simulink model "testBeam"  (R2014a)
settings: Solver=ode23t  StartTime=0.0  StopTime=100  MaxStep=1  RelTol=1e-3  AbsTol=1e-3
PreLoadFcn:
  | K = 1e6;
  | C = 1e4;
  | L = 1;
  | w = 0.5;
  | d = 0.1;
undefined symbols (not defined in the file): X, Y, Z
libraries: beamLib x25, sm_lib x7, nesl_utility x3, simulink x1
settings Model: Creator=grouleau  LastModifiedBy=grouleau
settings SolverCC: MaxConsecutiveZCs=100  SolverJacobianMethodControl=SparsePerturbation  ZeroCrossAlgorithm=Adaptive
settings DebuggingCC: UnderspecifiedInitializationDetection=Classic  ParameterPrecisionLossMsg=none
settings SimscapeCC: SimscapeLogType=all  SimscapeLogSimulationStatistics=on  SimscapeLogLimitData=off
settings ExplorerConfigSet: InternalSimMechanicsExplorerSettings="<ExplorerConfiguration><canonicalview>default</canonicalview><AnimationSetting><BasePlaybackSpeed>1.0</BasePlaybackSpeed><PlaybackSpeedFactor>8.0</PlaybackSpeedFactor></AnimationSetting><TilePanel><TileInfo><Tiles Columns=\"1\" Count=\"1\" Rows=\"1\"><Column Left=\"2\" Weight=\"1\"/><Column Left=\"828\"/><Row Top=\"2\" Weight=\"1\"/><Row Top=\"712\"/><Tile Height=\"1\" Width=\"1\" X=\"0\" Y=\"0\"/></Tiles></TileInfo><SceneInfo><SceneViewer><BGColor><R>0.60000002384185791</R><G>0.60000002384185791</G><B>0.60000002384185791</B></BGColor><Camera><Position><X>12.490758895874023</X><Y>0.67244863510131836</Y><Z>26.566392370959054</Z></Position><Center><X>12.490758895874023</X><Y>0.67244863510131836</Y><Z>0</Z></Center><Up><X>0</X><Y>1</Y><Z>-0</Z></Up><Left>-13.115296840667725</Left><Right>13.115296840667725</Right><Bottom>-0.91037138700485232</Bottom><Top>0.91037138700485232</Top></Camera></SceneViewer></SceneInfo></TilePanel></ExplorerConfiguration>"

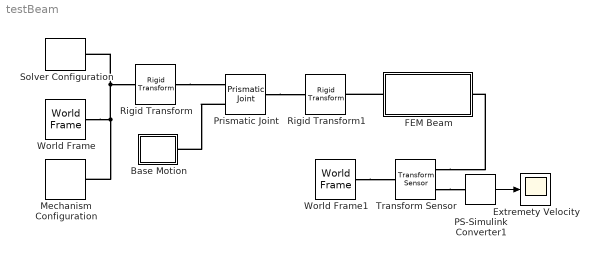
== system testBeam ==
  Base Motion : Subsystem
  Extremety Velocity : Scope
      settings: YMin=-50  YMax=50
  FEM Beam : Subsystem  mask{K=K, C=C, L=L, w=w, d=d, N=25}
      mask prompts: K "Stiffness"; C "Damping"; L "Length"; w "width"; d "Tickness"; N "Numbe rof elements"
      mask init:
      | blk = gcb;
      | 
      | blks = find_system(blk,'lookundermasks','all',...
      |     'followlinks','on',...
      |     'findall','on');
      | 
      | [hB, hF] = delete_beam_segments(blks);
      | add_beam_segments(blk,hB,hF,N)
  Mechanism Configuration : sm_lib/Utilities/Mechanism Configuration  UniformGravity=Constant  GravityVector=[0 0 -9.80665]*0  GravityUnits=m/s^2  LinearizationDelta=0.001  BlockFunction=simmechanics.library.utilities.mechanism_configuration
  PS-Simulink Converter1 : nesl_utility/PS-Simulink Converter  PhysicalDomain=network_engine_domain  SubClassName=ps_output  LeftPortType=input  RightPortType=output  PseudoPeriodic=off  Frequencies=[]  Unit=1  AffineConversion=off
  Prismatic Joint : sm_lib/Joints/Prismatic Joint  SenseConstraintForce=off  SenseConstraintForceX=off  SenseConstraintForceY=off  SenseConstraintForceZ=off  SenseConstraintTorque=off  SenseConstraintTorqueX=off  SenseConstraintTorqueY=off  SenseConstraintTorqueZ=off  SenseTotalForce=off  SenseTotalForceX=off  SenseTotalForceY=off  SenseTotalForceZ=off  SenseTotalTorque=off  SenseTotalTorqueX=off  SenseTotalTorqueY=off  SenseTotalTorqueZ=off  CompositeWrenchDir=FollowerOnBase  CompositeWrenchFrame=BaseFrame  EquilibriumPosition=0  EquilibriumPositionUnits=m  SpringStiffness=0  SpringStiffnessUnits=N/m  DampingCoefficient=0  DampingCoefficientUnits=N/(m/s)  TorqueActuationMode=ComputedTorque  MotionActuationMode=InputMotion  SensePosition=off  SenseVelocity=off  SenseAcceleration=off  SenseTorqueForce=off  PositionTargetValue=0  PositionTargetValueUnits=m  PositionTargetSpecify=off  PositionTargetPriority=High  VelocityTargetValue=0  VelocityTargetValueUnits=m/s  VelocityTargetSpecify=off  VelocityTargetPriority=High  BlockFunction=simmechanics.library.joints.prismatic_joint
  Rigid Transform : sm_lib/Frames and Transforms/Rigid Transform  TranslationMethod=None  TranslationLengthUnit=m  TranslationStandardAxis=+Z  TranslationStandardOffset=0  TranslationCartesianOffset=[0 0 0]  TranslationROffset=0  TranslationROffsetUnits=m  TranslationZOffset=0  TranslationZOffsetUnits=m  TranslationThetaOffset=0  TranslationThetaOffsetUnits=deg  RotationMethod=StandardAxis  RotationAngleUnits=deg  RotationStandardAxis=+X  RotationAngle=-90  RotationArbitraryAxis=[0 0 1]  FollAlignAxisA=+X  BaseAlignAxisA=+Y  FollAlignAxisB=+Y  BaseAlignAxisB=+Z  BlockFunction=simmechanics.library.frames_transforms.rigid_transform
  Rigid Transform1 : sm_lib/Frames and Transforms/Rigid Transform  TranslationMethod=None  TranslationLengthUnit=m  TranslationStandardAxis=+Z  TranslationStandardOffset=0  TranslationCartesianOffset=[0 0 0]  TranslationROffset=0  TranslationROffsetUnits=m  TranslationZOffset=0  TranslationZOffsetUnits=m  TranslationThetaOffset=0  TranslationThetaOffsetUnits=deg  RotationMethod=StandardAxis  RotationAngleUnits=deg  RotationStandardAxis=+X  RotationAngle=-90  RotationArbitraryAxis=[0 0 1]  FollAlignAxisA=+X  BaseAlignAxisA=+Y  FollAlignAxisB=+Y  BaseAlignAxisB=+Z  BlockFunction=simmechanics.library.frames_transforms.rigid_transform
  Solver Configuration : nesl_utility/Solver Configuration  PhysicalDomain=network_engine_domain  SubClassName=solver  LeftPortType=input  RightPortType=generic  Accelerate=off  Tones=[]  Harmonics=[]  SimulateNoise=off  Profile=off  UseLocalSampling=off  EnableSwitchedLinearOptims=on  FrequencyDomain=off  UseCCode=off  RelTol=0.001  AbsTol=1e-06  MinStep=1e-09  ToWorkspace=off  DoDC=off  ResidualTolerance=1e-09  UseLocalSolver=off  LocalSolverChoice=NE_BACKWARD_EULER_ADVANCER  LocalSolverSampleTime=0.001  DoFixedCost=off  MaxNonlinIter=3  MaxModeIter=2  LinearAlgebra=Sparse  DelaysMemoryBudget=1024  AutomaticFiltering=on  FilteringTimeConstant=0.001
  Transform Sensor : sm_lib/Frames and Transforms/Transform Sensor  MeasurementFrame=World  SenseAngle=off  SenseAxis=off  SenseAngle1=off  SenseAngle2=off  SenseAngle3=off  SenseQ=off  SenseR=off  SenseOmegaX=off  SenseOmegaY=off  SenseOmegaZ=off  SenseOmega1=off  SenseOmega2=off  SenseOmega3=off  SenseQDot=off  SenseRDot=off  SenseAlphaX=off  SenseAlphaY=off  SenseAlphaZ=off  SenseAlpha1=off  SenseAlpha2=off  SenseAlpha3=off  SenseQDDot=off  SenseRDDot=off  SenseX=off  SenseY=off  SenseZ=off  SenseRad=off  SenseAzim=off  SenseDist=off  SenseInc=off  SenseXDot=off  SenseYDot=on  SenseZDot=off  SenseRadDot=off  SenseAzimDot=off  SenseDistDot=off  SenseIncDot=off  SenseXDDot=off  SenseYDDot=off  SenseZDDot=off  SenseRadDDot=off  SenseAzimDDot=off  SenseDistDDot=off  SenseIncDDot=off  BlockFunction=simmechanics.library.frames_transforms.transform_sensor
  World Frame : sm_lib/Frames and Transforms/World Frame  BlockFunction=simmechanics.library.frames_transforms.world_frame
  World Frame1 : sm_lib/Frames and Transforms/World Frame  BlockFunction=simmechanics.library.frames_transforms.world_frame
  wires:
  PS-Simulink Converter1/1 -> Extremety Velocity/1
  connections:
  World Frame/RConn1 -- Solver Configuration/RConn1 -- Rigid Transform/LConn1 -- Mechanism Configuration/RConn1
  Transform Sensor/RConn2 -- PS-Simulink Converter1/LConn1
  Prismatic Joint/RConn1 -- Rigid Transform1/LConn1
  FEM Beam/LConn1 -- Rigid Transform1/RConn1
  Rigid Transform/RConn1 -- Prismatic Joint/LConn1
  World Frame1/RConn1 -- Transform Sensor/LConn1
  Transform Sensor/RConn1 -- FEM Beam/RConn1
  Prismatic Joint/LConn2 -- Base Motion/RConn1

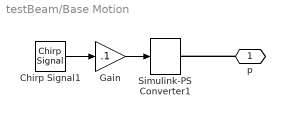
== system testBeam/Base Motion ==
  Chirp Signal1 : simulink/Sources/Chirp Signal  f1=.2  T=100  f2=2
  Gain : Gain  Gain=.1
  Simulink-PS Converter1 : nesl_utility/Simulink-PS Converter  PhysicalDomain=network_engine_domain  SubClassName=ps_input  LeftPortType=input  RightPortType=output  PseudoPeriodic=off  Frequencies=[]  NoiseDistribution=none  NoiseParameters=[]  Unit=1  AffineConversion=off  InputFiltering=on  SimscapeFilterOrder=2  InputFilterTimeConstant=0.001  UdotUserProvided=1
  p : PMIOPort  Port=1  Side=Right
  wires:
  Chirp Signal1/1 -> Gain/1
  Gain/1 -> Simulink-PS Converter1/1
  connections:
  p/RConn1 -- Simulink-PS Converter1/RConn1

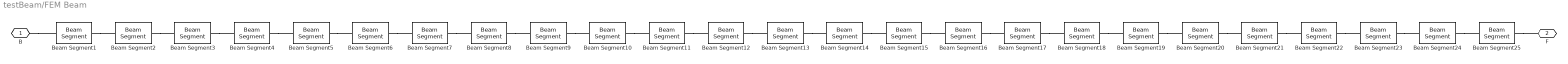
== system testBeam/FEM Beam ==
  Beam Segment{1..25} (25 alike) : beamLib/Beam Segment  K=K  C=C  L=L  w=w  d=d
  B : PMIOPort  Port=1  Side=Left
  F : PMIOPort  Port=2  Side=Right
  connections:
  B/RConn1 -- Beam Segment1/LConn1
  Beam Segment1/RConn1 -- Beam Segment2/LConn1
  Beam Segment2/RConn1 -- Beam Segment3/LConn1
  Beam Segment3/RConn1 -- Beam Segment4/LConn1
  Beam Segment4/RConn1 -- Beam Segment5/LConn1
  Beam Segment5/RConn1 -- Beam Segment6/LConn1
  Beam Segment6/RConn1 -- Beam Segment7/LConn1
  Beam Segment7/RConn1 -- Beam Segment8/LConn1
  Beam Segment8/RConn1 -- Beam Segment9/LConn1
  Beam Segment9/RConn1 -- Beam Segment10/LConn1
  Beam Segment10/RConn1 -- Beam Segment11/LConn1
  Beam Segment11/RConn1 -- Beam Segment12/LConn1
  Beam Segment12/RConn1 -- Beam Segment13/LConn1
  Beam Segment13/RConn1 -- Beam Segment14/LConn1
  Beam Segment14/RConn1 -- Beam Segment15/LConn1
  Beam Segment15/RConn1 -- Beam Segment16/LConn1
  Beam Segment16/RConn1 -- Beam Segment17/LConn1
  Beam Segment17/RConn1 -- Beam Segment18/LConn1
  Beam Segment18/RConn1 -- Beam Segment19/LConn1
  Beam Segment19/RConn1 -- Beam Segment20/LConn1
  Beam Segment20/RConn1 -- Beam Segment21/LConn1
  Beam Segment21/RConn1 -- Beam Segment22/LConn1
  Beam Segment22/RConn1 -- Beam Segment23/LConn1
  Beam Segment23/RConn1 -- Beam Segment24/LConn1
  Beam Segment24/RConn1 -- Beam Segment25/LConn1
  Beam Segment25/RConn1 -- F/RConn1
